simulink model "test2"  (R2015a)
settings: Solver=ode45  StartTime=0.0  StopTime=100000  RelTol=1e-3
InitFcn:
  | %% DSPBuilder Start
  | alt_dspbuilder_update_model(bdroot)
  | %% DSPBuilder End
libraries: allblocks_alteradspbuilder2 x988
(part 1 of 12)
settings Model: Creator=ASUS  LastModifiedBy=ASUS

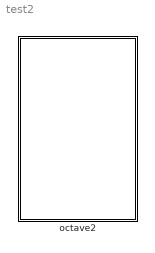
== system test2 ==
  octave2 : Subsystem

== system test2/octave2 ==
  AltBus : allblocks_alteradspbuilder2/AltBus  BusType=Unsigned Integer  bwl=128  bwr=0  saturate=off  floatingPointInput=on  floatingPointOutput=on  logOutputs=off  logFile=C:\Users\ASUS\Desktop\sift_fpga_final\Octave_2\tb_test2\test2_octave2_AltBus.fixedpointlog
  AltBus1 : allblocks_alteradspbuilder2/AltBus  BusType=Unsigned Fractional  bwl=8  bwr=16  saturate=off  floatingPointInput=on  floatingPointOutput=on  logOutputs=off  logFile=C:\Users\ASUS\Desktop\sift_fpga_final\Octave_2\tb_test2\test2_octave2_AltBus1.fixedpointlog
  AltBus2 : allblocks_alteradspbuilder2/AltBus  BusType=Unsigned Integer  bwl=10  bwr=16  saturate=off  floatingPointInput=on  floatingPointOutput=on  logOutputs=off  logFile=C:\Users\ASUS\Desktop\sift_fpga_final\Octave_2\tb_test2\test2_octave2_AltBus2.fixedpointlog
  AltBus3 : allblocks_alteradspbuilder2/AltBus  BusType=Unsigned Integer  bwl=8  bwr=0  saturate=off  floatingPointInput=on  floatingPointOutput=on  logOutputs=off  logFile=C:\Users\ASUS\Desktop\sift_fpga_final\Octave_2\tb_test2\test2_octave2_AltBus3.fixedpointlog
  Bus_Concatenation : Subsystem
  From Workspace : FromWorkspace  VariableName=pixel_in  SampleTime=0
  From Workspace1 : FromWorkspace  VariableName=valid_in  SampleTime=0
  From Workspace2 : FromWorkspace  VariableName=sof_in  SampleTime=0
  From Workspace3 : FromWorkspace  VariableName=eof_in  SampleTime=0
  GradOrien : Subsystem
  Line_buff_11x11 : Subsystem
  descriptor : Subsystem
  hist_bin : Subsystem
  scale_space : Subsystem
  sink_validIn : allblocks_alteradspbuilder2/Input  iofile=C:\Users\ASUS\Desktop\sift_fpga_final\Octave_2\tb_test2\test2_octave2_sink%5FvalidIn.salt  BusType=Single Bit  bwl=8  bwr=0  SpecifyClock=off  PORTTYPE=Input  externalType=Inferred  allowFloatingPointOverride=on  logOutputs=off
  sink_validIn1 : allblocks_alteradspbuilder2/Input  iofile=C:\Users\ASUS\Desktop\sift_fpga_final\Octave_2\tb_test2\test2_octave2_sink%5FvalidIn1.salt  BusType=Single Bit  bwl=8  bwr=0  SpecifyClock=off  PORTTYPE=Input  externalType=Inferred  allowFloatingPointOverride=on  logOutputs=off
  sink_validIn2 : allblocks_alteradspbuilder2/Input  iofile=C:\Users\ASUS\Desktop\sift_fpga_final\Octave_2\tb_test2\test2_octave2_sink%5FvalidIn2.salt  BusType=Single Bit  bwl=8  bwr=0  SpecifyClock=off  PORTTYPE=Input  externalType=Inferred  allowFloatingPointOverride=on  logOutputs=off
  sink_validIn3 : allblocks_alteradspbuilder2/Input  iofile=C:\Users\ASUS\Desktop\sift_fpga_final\Octave_2\tb_test2\test2_octave2_sink%5FvalidIn3.salt  BusType=Unsigned Integer  bwl=8  bwr=0  SpecifyClock=off  PORTTYPE=Input  externalType=Inferred  allowFloatingPointOverride=on  logOutputs=off
  wires:
  GradOrien/1(m_xy) -> AltBus2/1
  hist_bin/6(hist_bin6_out) -> Bus_Concatenation/6(bin6_in)
  hist_bin/8(hist_bin8_out) -> Bus_Concatenation/8(bin8_in)
  [valid_in] -> scale_space/2(valid_in)
  scale_space/1(scale2) -> AltBus1/1
  [valid_in] -> GradOrien/2(clken)
  [pixel_in] -> scale_space/1(data_in)
  [valid_in] -> hist_bin/3(clken)
  GradOrien/2(orien) -> AltBus3/1
  hist_bin/7(hist_bin7_out) -> Bus_Concatenation/7(bin_in)
  Line_buff_11x11/9(Out1010) -> descriptor/9(data_in1010)
  Line_buff_11x11/1(Out00) -> descriptor/1(data_in00)
  Line_buff_11x11/6(Out510) -> descriptor/6(data_in510)
  Line_buff_11x11/3(Out010) -> descriptor/3(data_in010)
  Line_buff_11x11/7(Out100) -> descriptor/7(data_in100)
  hist_bin/5(hist_bin5_out) -> Bus_Concatenation/5(bin5_in)
  hist_bin/3(hist_bin3_out) -> Bus_Concatenation/3(biin3_in)
  hist_bin/2(hist_bin2_out) -> Bus_Concatenation/2(bin2_in)
  Line_buff_11x11/2(Out05) -> descriptor/2(data_in05)
  hist_bin/1(hist_bin1_out) -> Bus_Concatenation/1(bin1_in)
  [valid_in] -> Line_buff_11x11/2(clken)
  hist_bin/4(hist_bin4_out) -> Bus_Concatenation/4(bin4_in)
  Line_buff_11x11/4(Out50) -> descriptor/4(data_in50)
  Line_buff_11x11/5(Out55) -> descriptor/5(data_in55)
  Bus_Concatenation/1(hist_bin) -> AltBus/1
  Line_buff_11x11/8(Out105) -> descriptor/8(data_in105)
  From Workspace2/1 -> sink_validIn1/1
  From Workspace/1 -> sink_validIn3/1
  From Workspace3/1 -> sink_validIn/1
  From Workspace1/1 -> sink_validIn2/1
  sink_validIn/1 -> [eof_in]
  sink_validIn1/1 -> [sof_in]
  sink_validIn2/1 -> [valid_in]
  sink_validIn3/1 -> [pixel_in]
  AltBus/1 -> Line_buff_11x11/1(dataIn)
  AltBus1/1 -> GradOrien/1(data_in)
  AltBus2/1 -> hist_bin/1(m_xy_In)
  AltBus3/1 -> hist_bin/2(orien_In)

== system test2/octave2/Bus_Concatenation ==
  bin1_in : Inport
  bin2_in : Inport  Port=2
  biin3_in : Inport  Port=3
  bin4_in : Inport  Port=4
  bin5_in : Inport  Port=5
  bin6_in : Inport  Port=6
  bin_in : Inport  Port=7
  bin8_in : Inport  Port=8
  Bus Concatenation{,1..3} (4 alike) : allblocks_alteradspbuilder2/Bus Concatenation  isSigned=off  awidth=16  bwidth=16  pipeline_display=0
  Bus Concatenation7 : allblocks_alteradspbuilder2/Bus Concatenation  isSigned=off  awidth=32  bwidth=32  pipeline_display=0
  Bus Concatenation8 : allblocks_alteradspbuilder2/Bus Concatenation  isSigned=off  awidth=32  bwidth=32  pipeline_display=0
  Bus Concatenation9 : allblocks_alteradspbuilder2/Bus Concatenation  isSigned=off  awidth=64  bwidth=64  pipeline_display=0
  To Workspace : ToWorkspace  VariableName=bin1  SaveFormat=Timeseries  SampleTime=-1
  hist_bin : Outport
  wires:
  bin1_in/1 -> [bin1]
  bin2_in/1 -> [bin2]
  biin3_in/1 -> [bin3]
  bin4_in/1 -> [bin4]
  bin5_in/1 -> [bin5]
  bin6_in/1 -> [bin6]
  bin_in/1 -> [bin7]
  bin8_in/1 -> [bin8]
  Bus Concatenation/1 -> Bus Concatenation8/2
  [bin6] -> Bus Concatenation1/2
  Bus Concatenation1/1 -> Bus Concatenation8/1
  [bin8] -> Bus Concatenation/2
  [bin5] -> Bus Concatenation1/1
  [bin7] -> Bus Concatenation/1
  Bus Concatenation9/1 -> To Workspace/1, hist_bin/1
  [bin4] -> Bus Concatenation2/2
  [bin3] -> Bus Concatenation2/1
  [bin2] -> Bus Concatenation3/2
  [bin1] -> Bus Concatenation3/1
  Bus Concatenation3/1 -> Bus Concatenation7/1
  Bus Concatenation2/1 -> Bus Concatenation7/2
  Bus Concatenation7/1 -> Bus Concatenation9/1
  Bus Concatenation8/1 -> Bus Concatenation9/2

== system test2/octave2/GradOrien ==
  data_in : Inport
  clken : Inport  Port=2
  lineBuff_3x3 : Subsystem
  sub_GradOrian : Subsystem
  m_xy : Outport
  orien : Outport  Port=2
  wires:
  sub_GradOrian/1(orien) -> orien/1
  clken/1 -> sub_GradOrian/5(clken), lineBuff_3x3/2(clken)
  data_in/1 -> lineBuff_3x3/1(dataIn)
  sub_GradOrian/2(m_xy) -> m_xy/1
  lineBuff_3x3/1(Out01) -> sub_GradOrian/1(L_y_add_1)
  lineBuff_3x3/4(Out21) -> sub_GradOrian/4(L_y_sub_1)
  lineBuff_3x3/3(Out12) -> sub_GradOrian/3(L_x_sub_1)
  lineBuff_3x3/2(Out10) -> sub_GradOrian/2(L_x_add_1)

== system test2/octave2/Line_buff_11x11 ==
  dataIn : Inport
  clken : Inport  Port=2
  Memory Delay1 : allblocks_alteradspbuilder2/Memory Delay  BusType=Unsigned Integer  bwl=128  bwr=0  pipeline=1  pipeline_display=1  ram_type=AUTO  use_ena=on  use_sclr=off  allowFloatingPointOverride=on  logOutputs=off  logFile=C:\Users\ASUS\Desktop\sift_fpga_final\Octave_2\tb_test2\test2_octave2_Line%5Fbuff%5F11x11_Memory+Delay1.fixedpointlog
  Memory Delay11 : allblocks_alteradspbuilder2/Memory Delay  BusType=Unsigned Integer  bwl=128  bwr=0  pipeline=630  pipeline_display=630  ram_type=AUTO  use_ena=on  use_sclr=off  allowFloatingPointOverride=on  logOutputs=off  logFile=C:\Users\ASUS\Desktop\sift_fpga_final\Octave_2\tb_test2\test2_octave2_Line%5Fbuff%5F11x11_Memory+Delay11.fixedpointlog
  Memory Delay12 : allblocks_alteradspbuilder2/Memory Delay  BusType=Unsigned Integer  bwl=128  bwr=0  pipeline=5  pipeline_display=5  ram_type=AUTO  use_ena=on  use_sclr=off  allowFloatingPointOverride=on  logOutputs=off  logFile=C:\Users\ASUS\Desktop\sift_fpga_final\Octave_2\tb_test2\test2_octave2_Line%5Fbuff%5F11x11_Memory+Delay12.fixedpointlog
  Memory Delay13 : allblocks_alteradspbuilder2/Memory Delay  BusType=Unsigned Integer  bwl=128  bwr=0  pipeline=5  pipeline_display=5  ram_type=AUTO  use_ena=on  use_sclr=off  allowFloatingPointOverride=on  logOutputs=off  logFile=C:\Users\ASUS\Desktop\sift_fpga_final\Octave_2\tb_test2\test2_octave2_Line%5Fbuff%5F11x11_Memory+Delay13.fixedpointlog
  Memory Delay15 : allblocks_alteradspbuilder2/Memory Delay  BusType=Unsigned Integer  bwl=128  bwr=0  pipeline=630  pipeline_display=630  ram_type=AUTO  use_ena=on  use_sclr=off  allowFloatingPointOverride=on  logOutputs=off  logFile=C:\Users\ASUS\Desktop\sift_fpga_final\Octave_2\tb_test2\test2_octave2_Line%5Fbuff%5F11x11_Memory+Delay15.fixedpointlog
  Memory Delay16 : allblocks_alteradspbuilder2/Memory Delay  BusType=Unsigned Integer  bwl=128  bwr=0  pipeline=5  pipeline_display=5  ram_type=AUTO  use_ena=on  use_sclr=off  allowFloatingPointOverride=on  logOutputs=off  logFile=C:\Users\ASUS\Desktop\sift_fpga_final\Octave_2\tb_test2\test2_octave2_Line%5Fbuff%5F11x11_Memory+Delay16.fixedpointlog
  Memory Delay17 : allblocks_alteradspbuilder2/Memory Delay  BusType=Unsigned Integer  bwl=128  bwr=0  pipeline=5  pipeline_display=5  ram_type=AUTO  use_ena=on  use_sclr=off  allowFloatingPointOverride=on  logOutputs=off  logFile=C:\Users\ASUS\Desktop\sift_fpga_final\Octave_2\tb_test2\test2_octave2_Line%5Fbuff%5F11x11_Memory+Delay17.fixedpointlog
  Memory Delay18 : allblocks_alteradspbuilder2/Memory Delay  BusType=Unsigned Integer  bwl=128  bwr=0  pipeline=640*4  pipeline_display=2560  ram_type=AUTO  use_ena=on  use_sclr=off  allowFloatingPointOverride=on  logOutputs=off  logFile=C:\Users\ASUS\Desktop\sift_fpga_final\Octave_2\tb_test2\test2_octave2_Line%5Fbuff%5F11x11_Memory+Delay18.fixedpointlog
  Memory Delay5 : allblocks_alteradspbuilder2/Memory Delay  BusType=Unsigned Integer  bwl=128  bwr=0  pipeline=5  pipeline_display=5  ram_type=AUTO  use_ena=on  use_sclr=off  allowFloatingPointOverride=on  logOutputs=off  logFile=C:\Users\ASUS\Desktop\sift_fpga_final\Octave_2\tb_test2\test2_octave2_Line%5Fbuff%5F11x11_Memory+Delay5.fixedpointlog
  Memory Delay6 : allblocks_alteradspbuilder2/Memory Delay  BusType=Unsigned Integer  bwl=128  bwr=0  pipeline=5  pipeline_display=5  ram_type=AUTO  use_ena=on  use_sclr=off  allowFloatingPointOverride=on  logOutputs=off  logFile=C:\Users\ASUS\Desktop\sift_fpga_final\Octave_2\tb_test2\test2_octave2_Line%5Fbuff%5F11x11_Memory+Delay6.fixedpointlog
  Memory Delay7 : allblocks_alteradspbuilder2/Memory Delay  BusType=Unsigned Integer  bwl=128  bwr=0  pipeline=640*4  pipeline_display=2560  ram_type=AUTO  use_ena=on  use_sclr=off  allowFloatingPointOverride=on  logOutputs=off  logFile=C:\Users\ASUS\Desktop\sift_fpga_final\Octave_2\tb_test2\test2_octave2_Line%5Fbuff%5F11x11_Memory+Delay7.fixedpointlog
  Out00 : Outport
  Out05 : Outport  Port=2
  Out010 : Outport  Port=3
  Out50 : Outport  Port=4
  Out55 : Outport  Port=5
  Out510 : Outport  Port=6
  Out100 : Outport  Port=7
  Out105 : Outport  Port=8
  Out1010 : Outport  Port=9
  wires:
  [clken] -> Memory Delay11/2
  [clken] -> Memory Delay17/2
  [clken] -> Memory Delay6/2
  Memory Delay6/1 -> [data_010], Memory Delay7/1
  [clken] -> Memory Delay18/2
  Memory Delay18/1 -> Memory Delay15/1
  Memory Delay13/1 -> Memory Delay18/1, [data_510]
  [clken] -> Memory Delay15/2
  [clken] -> Memory Delay16/2
  Memory Delay17/1 -> [data_1010]
  Memory Delay16/1 -> Memory Delay17/1, [data_105]
  Memory Delay15/1 -> Memory Delay16/1, [data_100]
  [clken] -> Memory Delay7/2
  [clken] -> Memory Delay12/2
  Memory Delay11/1 -> Memory Delay12/1, [data_50]
  Memory Delay12/1 -> Memory Delay13/1, [data_55]
  Memory Delay7/1 -> Memory Delay11/1
  [clken] -> Memory Delay13/2
  [data_55] -> Out55/1
  [data_010] -> Out010/1
  [data_05] -> Out05/1
  clken/1 -> [clken]
  [data_00] -> Out00/1
  [data_50] -> Out50/1
  [data_100] -> Out100/1
  [data_510] -> Out510/1
  [data_1010] -> Out1010/1
  dataIn/1 -> [data_in]
  [data_105] -> Out105/1
  [clken] -> Memory Delay5/2
  Memory Delay1/1 -> Memory Delay5/1, [data_00]
  [clken] -> Memory Delay1/2
  [data_in] -> Memory Delay1/1
  Memory Delay5/1 -> Memory Delay6/1, [data_05]

== system test2/octave2/descriptor ==
  data_in00 : Inport
  data_in05 : Inport  Port=2
  data_in010 : Inport  Port=3
  data_in50 : Inport  Port=4
  data_in55 : Inport  Port=5
  data_in510 : Inport  Port=6
  data_in100 : Inport  Port=7
  data_in105 : Inport  Port=8
  data_in1010 : Inport  Port=9
  AltBus : allblocks_alteradspbuilder2/AltBus  BusType=Unsigned Integer  bwl=128*9  bwr=0  saturate=off  floatingPointInput=on  floatingPointOutput=on  logOutputs=off  logFile=C:\Users\ASUS\Desktop\sift_fpga_final\Octave_2\tb_test2\test2_octave2_descriptor_AltBus.fixedpointlog
  BusSplitter : Subsystem
  Multiplexer3 : allblocks_alteradspbuilder2/Multiplexer  numInputs=8  pipeline=0  oneHot=off  pipeline_display=0  use_ena=off  use_aclr=off  allowFloatingPointOverride=on  logOutputs=off  logFile=C:\Users\ASUS\Desktop\sift_fpga_final\Octave_2\tb_test2\test2_octave2_descriptor_Multiplexer3.fixedpointlog
  To Workspace1 : ToWorkspace  VariableName=descriptor  SaveFormat=Timeseries  SampleTime=-1
  To Workspace4 : ToWorkspace  VariableName=bin55  SaveFormat=Timeseries  SampleTime=-1
  To Workspace5 : ToWorkspace  VariableName=binmax  SaveFormat=Timeseries  SampleTime=-1
  descriptor : Subsystem
  findMax : Subsystem
  wires:
  [hist_105] -> descriptor/8(data_in8)
  [hist_100] -> descriptor/7(data_in7)
  [hist_510] -> descriptor/6(data_in6)
  [hist_55] -> descriptor/5(data_in5)
  [hist_1010] -> descriptor/9(data_in9)
  descriptor/1(descriptor1) -> Multiplexer3/2
  [hist_05] -> descriptor/2(data_in2)
  [hist_010] -> descriptor/3(data_in3)
  [hist_50] -> descriptor/4(data_in4)
  descriptor/5(descriptor5) -> Multiplexer3/6
  descriptor/4(descriptor4) -> Multiplexer3/5
  [hist_00] -> descriptor/1(data_in1)
  descriptor/7(descriptor7) -> Multiplexer3/8
  descriptor/8(descriptor8) -> Multiplexer3/9
  descriptor/2(descriptor2) -> Multiplexer3/3
  descriptor/3(descriptor3) -> Multiplexer3/4
  descriptor/6(descriptor6) -> Multiplexer3/7
  BusSplitter/3(bin3) -> findMax/3(bin3)
  data_in00/1 -> [hist_00]
  data_in50/1 -> [hist_50]
  BusSplitter/1(bin1) -> findMax/1(bin1)
  data_in100/1 -> [hist_100]
  data_in010/1 -> [hist_010]
  data_in105/1 -> [hist_105]
  [hist_55] -> To Workspace4/1, BusSplitter/1(data_in)
  data_in510/1 -> [hist_510]
  data_in1010/1 -> [hist_1010]
  BusSplitter/8(bin8) -> findMax/8(bin8)
  data_in55/1 -> [hist_55]
  BusSplitter/4(bin4) -> findMax/4(bin4)
  BusSplitter/2(bin2) -> findMax/2(bin2)
  data_in05/1 -> [hist_05]
  BusSplitter/5(bin5) -> findMax/5(bin5)
  BusSplitter/7(bin7) -> findMax/7(bin7)
  BusSplitter/6(bin6) -> findMax/6(bin6)
  AltBus/1 -> [descriptor]
  findMax/1(bin_max) -> To Workspace5/1, Multiplexer3/1
  Multiplexer3/1 -> To Workspace1/1, AltBus/1

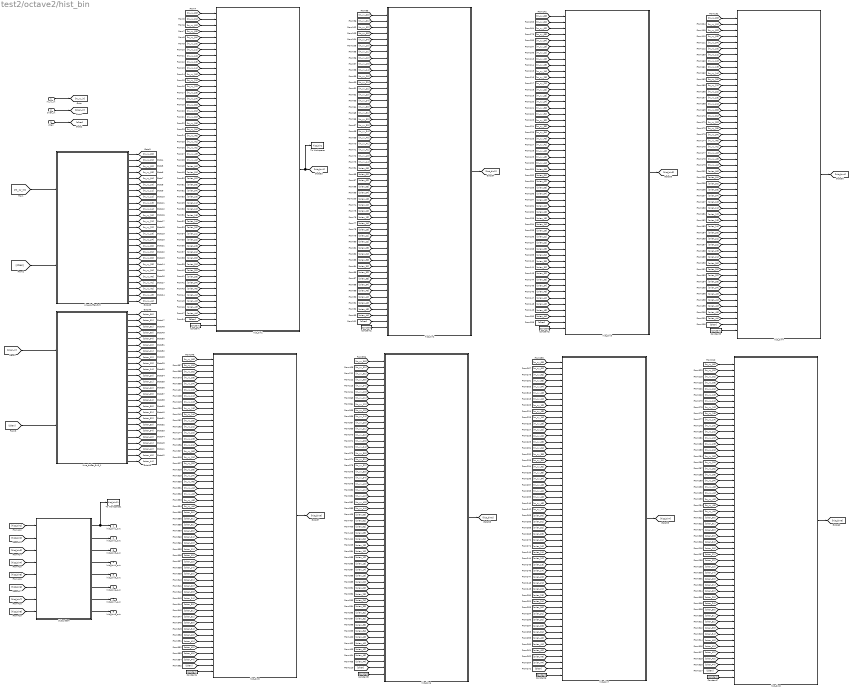
== system test2/octave2/hist_bin ==
  m_xy_In : Inport
  orien_In : Inport  Port=2
  clken : Inport  Port=3
  Constant : allblocks_alteradspbuilder2/Constant  mask_cst=1  BusType=Unsigned Integer  bwl=8  bwr=0  roundMode=Truncate  satMode=Wrap  SpecifyClock=off  allowFloatingPointOverride=on  logOutputs=off  logFile=C:\Users\ASUS\Desktop\sift_fpga_final\Octave_2\tb_test2\test2_octave2_hist%5Fbin_Constant.fixedpointlog
  Constant1 : allblocks_alteradspbuilder2/Constant  mask_cst=2  BusType=Unsigned Integer  bwl=8  bwr=0  roundMode=Truncate  satMode=Wrap  SpecifyClock=off  allowFloatingPointOverride=on  logOutputs=off  logFile=C:\Users\ASUS\Desktop\sift_fpga_final\Octave_2\tb_test2\test2_octave2_hist%5Fbin_Constant1.fixedpointlog
  Constant2 : allblocks_alteradspbuilder2/Constant  mask_cst=3  BusType=Unsigned Integer  bwl=8  bwr=0  roundMode=Truncate  satMode=Wrap  SpecifyClock=off  allowFloatingPointOverride=on  logOutputs=off  logFile=C:\Users\ASUS\Desktop\sift_fpga_final\Octave_2\tb_test2\test2_octave2_hist%5Fbin_Constant2.fixedpointlog
  Constant3 : allblocks_alteradspbuilder2/Constant  mask_cst=4  BusType=Unsigned Integer  bwl=8  bwr=0  roundMode=Truncate  satMode=Wrap  SpecifyClock=off  allowFloatingPointOverride=on  logOutputs=off  logFile=C:\Users\ASUS\Desktop\sift_fpga_final\Octave_2\tb_test2\test2_octave2_hist%5Fbin_Constant3.fixedpointlog
  Constant4 : allblocks_alteradspbuilder2/Constant  mask_cst=5  BusType=Unsigned Integer  bwl=8  bwr=0  roundMode=Truncate  satMode=Wrap  SpecifyClock=off  allowFloatingPointOverride=on  logOutputs=off  logFile=C:\Users\ASUS\Desktop\sift_fpga_final\Octave_2\tb_test2\test2_octave2_hist%5Fbin_Constant4.fixedpointlog
  Constant5 : allblocks_alteradspbuilder2/Constant  mask_cst=6  BusType=Unsigned Integer  bwl=8  bwr=0  roundMode=Truncate  satMode=Wrap  SpecifyClock=off  allowFloatingPointOverride=on  logOutputs=off  logFile=C:\Users\ASUS\Desktop\sift_fpga_final\Octave_2\tb_test2\test2_octave2_hist%5Fbin_Constant5.fixedpointlog
  Constant6 : allblocks_alteradspbuilder2/Constant  mask_cst=7  BusType=Unsigned Integer  bwl=8  bwr=0  roundMode=Truncate  satMode=Wrap  SpecifyClock=off  allowFloatingPointOverride=on  logOutputs=off  logFile=C:\Users\ASUS\Desktop\sift_fpga_final\Octave_2\tb_test2\test2_octave2_hist%5Fbin_Constant6.fixedpointlog
  Constant7 : allblocks_alteradspbuilder2/Constant  mask_cst=8  BusType=Unsigned Integer  bwl=8  bwr=0  roundMode=Truncate  satMode=Wrap  SpecifyClock=off  allowFloatingPointOverride=on  logOutputs=off  logFile=C:\Users\ASUS\Desktop\sift_fpga_final\Octave_2\tb_test2\test2_octave2_hist%5Fbin_Constant7.fixedpointlog
  Line_buffer_5x5 : Subsystem
  Line_buffer_5x5_1 : Subsystem
  Subsystem : Subsystem
  To Workspace : ToWorkspace  VariableName=hist_bin1  SaveFormat=Timeseries  SampleTime=-1
  To Workspace1 : ToWorkspace  VariableName=hist_bin11  SaveFormat=Timeseries  SampleTime=-1
  hist_bin1 : Subsystem
  hist_bin2 : Subsystem
  hist_bin3 : Subsystem
  hist_bin4 : Subsystem
  hist_bin5 : Subsystem
  hist_bin6 : Subsystem
  hist_bin7 : Subsystem
  hist_bin8 : Subsystem
  hist_bin1_out : Outport
  hist_bin2_out : Outport  Port=2
  hist_bin3_out : Outport  Port=3
  hist_bin4_out : Outport  Port=4
  hist_bin5_out : Outport  Port=5
  hist_bin6_out : Outport  Port=6
  hist_bin7_out : Outport  Port=7
  hist_bin8_out : Outport  Port=8
  wires:
  [hist_bin7] -> Subsystem/7(hist_in_bin7)
  [m_xy_in] -> Line_buffer_5x5/1(dataIn)
  [clken] -> Line_buffer_5x5/2(clken)
  [clken] -> Line_buffer_5x5_1/2(clken)
  [orien_in] -> Line_buffer_5x5_1/1(dataIn)
  clken/1 -> [clken]
  Line_buffer_5x5_1/21(Out40) -> [orien_40]
  Line_buffer_5x5_1/19(Out33) -> [orien_33]
  Line_buffer_5x5_1/8(Out12) -> [orien_12]
  Line_buffer_5x5_1/14(Out23) -> [orien_23]
  Line_buffer_5x5_1/18(Out32) -> [orien_32]
  Line_buffer_5x5_1/20(Out34) -> [orien_34]
  Line_buffer_5x5_1/2(Out01) -> [orien_01]
  Line_buffer_5x5_1/7(Out11) -> [orien_11]
  Line_buffer_5x5_1/11(Out20) -> [orien_20]
  Line_buffer_5x5_1/13(Out22) -> [orien_22]
  Line_buffer_5x5_1/17(Out31) -> [orien_31]
  Line_buffer_5x5_1/25(Out44) -> [orien_44]
  Line_buffer_5x5_1/3(Out02) -> [orien_02]
  Line_buffer_5x5_1/5(Out04) -> [orien_04]
  Line_buffer_5x5_1/23(Out42) -> [orien_42]
  Line_buffer_5x5_1/24(Out43) -> [orien_43]
  Line_buffer_5x5_1/6(Out10) -> [orien_10]
  Line_buffer_5x5_1/1(Out00) -> [orien_00]
  Line_buffer_5x5_1/22(Out41) -> [orien_41]
  Line_buffer_5x5_1/15(Out24) -> [orien_24]
  Line_buffer_5x5_1/4(Out03) -> [orien_03]
  Line_buffer_5x5_1/9(Out13) -> [orien_13]
  Line_buffer_5x5_1/10(Out14) -> [orien_14]
  Line_buffer_5x5_1/12(Out21) -> [orien_21]
  Line_buffer_5x5_1/16(Out30) -> [orien_30]
  Line_buffer_5x5/24(Out43) -> [m_xy_43]
  Line_buffer_5x5/21(Out40) -> [m_xy_40]
  Line_buffer_5x5/23(Out42) -> [m_xy_42]
  Line_buffer_5x5/22(Out41) -> [m_xy_41]
  Line_buffer_5x5/25(Out44) -> [m_xy_44]
  Line_buffer_5x5/12(Out21) -> [m_xy_21]
  Line_buffer_5x5/15(Out24) -> [m_xy_24]
  Line_buffer_5x5/19(Out33) -> [m_xy_33]
  Line_buffer_5x5/18(Out32) -> [m_xy_32]
  Line_buffer_5x5/13(Out22) -> [m_xy_22]
  Line_buffer_5x5/11(Out20) -> [m_xy_20]
  Line_buffer_5x5/16(Out30) -> [m_xy_30]
  Line_buffer_5x5/14(Out23) -> [m_xy_23]
  Line_buffer_5x5/17(Out31) -> [m_xy_31]
  Line_buffer_5x5/20(Out34) -> [m_xy_34]
  [hist_bin1] -> Subsystem/1(hist_in_bin1)
  Line_buffer_5x5/1(Out00) -> [m_xy_00]
  [m_xy_04] -> hist_bin1/5(Mxy_In04)
  Line_buffer_5x5/2(Out01) -> [m_xy_01]
  hist_bin1/1(bin_out) -> To Workspace/1, [hist_bin1]
  [m_xy_10] -> hist_bin1/6(Mxy_In10)
  Line_buffer_5x5/9(Out13) -> [m_xy_13]
  [m_xy_13] -> hist_bin1/9(Mxy_In13)
  Line_buffer_5x5/10(Out14) -> [m_xy_14]
  Line_buffer_5x5/6(Out10) -> [m_xy_10]
  Line_buffer_5x5/7(Out11) -> [m_xy_11]
  [m_xy_11] -> hist_bin1/7(Mxy_In11)
  [m_xy_12] -> hist_bin1/8(Mxy_In12)
  Line_buffer_5x5/8(Out12) -> [m_xy_12]
  [m_xy_14] -> hist_bin1/10(Mxy_In14)
  [m_xy_22] -> hist_bin1/13(Mxy_In22)
  [m_xy_40] -> hist_bin1/21(Mxy_In40)
  [m_xy_43] -> hist_bin1/24(Mxy_In43)
  [m_xy_42] -> hist_bin1/23(Mxy_In42)
  [m_xy_44] -> hist_bin1/25(Mxy_In44)
  [m_xy_24] -> hist_bin1/15(Mxy_In24)
  [m_xy_21] -> hist_bin1/12(Mxy_In21)
  [m_xy_20] -> hist_bin1/11(Mxy_In20)
  [m_xy_23] -> hist_bin1/14(Mxy_In23)
  [m_xy_41] -> hist_bin1/22(Mxy_In41)
  [m_xy_01] -> hist_bin1/2(Mxy_In01)
  Line_buffer_5x5/4(Out03) -> [m_xy_03]
  Line_buffer_5x5/5(Out04) -> [m_xy_04]
  Line_buffer_5x5/3(Out02) -> [m_xy_02]
  [m_xy_31] -> hist_bin1/17(Mxy_In31)
  [m_xy_30] -> hist_bin1/16(Mxy_In30)
  [m_xy_34] -> hist_bin1/20(Mxy_In34)
  [m_xy_33] -> hist_bin1/19(Mxy_In33)
  [m_xy_32] -> hist_bin1/18(Mxy_In32)
  [m_xy_03] -> hist_bin1/4(Mxy_In03)
  [m_xy_02] -> hist_bin1/3(Mxy_In02)
  [hist_bin3] -> Subsystem/3(hist_in_bin3)
  [hist_bin4] -> Subsystem/4(hist_in_bin4)
  [orien_10] -> hist_bin1/31(Orien_In10)
  [orien_42] -> hist_bin1/48(Orien_In42)
  [orien_01] -> hist_bin1/27(Orien_In01)
  [orien_20] -> hist_bin1/36(Orien_In20)
  [orien_31] -> hist_bin1/42(Orien_In31)
  [orien_33] -> hist_bin1/44(Orien_In33)
  [orien_21] -> hist_bin1/37(Orien_In21)
  [orien_24] -> hist_bin1/40(Orien_In24)
  [orien_03] -> hist_bin1/29(Orien_In03)
  [orien_30] -> hist_bin1/41(Orien_In30)
  [orien_12] -> hist_bin1/33(Orien_In12)
  [orien_23] -> hist_bin1/39(Orien_In23)
  [orien_32] -> hist_bin1/43(Orien_In32)
  [orien_41] -> hist_bin1/47(Orien_In41)
  [orien_43] -> hist_bin1/49(Orien_In43)
  [orien_02] -> hist_bin1/28(Orien_In02)
  [orien_00] -> hist_bin1/26(Orien_In00)
  [orien_11] -> hist_bin1/32(Orien_In11)
  [orien_34] -> hist_bin1/45(Orien_In34)
  [orien_22] -> hist_bin1/38(Orien_In22)
  [orien_04] -> hist_bin1/30(Orien_In04)
  [orien_14] -> hist_bin1/35(Orien_In14)
  [orien_44] -> hist_bin1/50(Orien_In44)
  [orien_13] -> hist_bin1/34(Orien_In13)
  [orien_40] -> hist_bin1/46(Orien_In40)
  [clken] -> hist_bin1/51(clken)
  Constant/1 -> hist_bin1/52(bin_in)
  [m_xy_02] -> hist_bin2/3(Mxy_In02)
  [m_xy_04] -> hist_bin2/5(Mxy_In04)
  [m_xy_10] -> hist_bin2/6(Mxy_In10)
  [m_xy_23] -> hist_bin2/14(Mxy_In23)
  [m_xy_31] -> hist_bin2/17(Mxy_In31)
  [m_xy_30] -> hist_bin2/16(Mxy_In30)
  [m_xy_12] -> hist_bin2/8(Mxy_In12)
  [m_xy_32] -> hist_bin2/18(Mxy_In32)
  [m_xy_13] -> hist_bin2/9(Mxy_In13)
  [m_xy_33] -> hist_bin2/19(Mxy_In33)
  [m_xy_41] -> hist_bin2/22(Mxy_In41)
  [m_xy_01] -> hist_bin2/2(Mxy_In01)
  [m_xy_14] -> hist_bin2/10(Mxy_In14)
  [m_xy_40] -> hist_bin2/21(Mxy_In40)
  [m_xy_43] -> hist_bin2/24(Mxy_In43)
  [m_xy_20] -> hist_bin2/11(Mxy_In20)
  [m_xy_22] -> hist_bin2/13(Mxy_In22)
  [m_xy_24] -> hist_bin2/15(Mxy_In24)
  [m_xy_34] -> hist_bin2/20(Mxy_In34)
  [m_xy_03] -> hist_bin2/4(Mxy_In03)
  [m_xy_00] -> hist_bin2/1(Mxy_In00)
  [m_xy_11] -> hist_bin2/7(Mxy_In11)
  [m_xy_21] -> hist_bin2/12(Mxy_In21)
  [orien_31] -> hist_bin2/42(Orien_In31)
  [orien_34] -> hist_bin2/45(Orien_In34)
  [m_xy_42] -> hist_bin2/23(Mxy_In42)
  [orien_01] -> hist_bin2/27(Orien_In01)
  [orien_00] -> hist_bin2/26(Orien_In00)
  [orien_04] -> hist_bin2/30(Orien_In04)
  [orien_13] -> hist_bin2/34(Orien_In13)
  [orien_20] -> hist_bin2/36(Orien_In20)
  [orien_24] -> hist_bin2/40(Orien_In24)
  [orien_33] -> hist_bin2/44(Orien_In33)
  [orien_32] -> hist_bin2/43(Orien_In32)
  [orien_41] -> hist_bin2/47(Orien_In41)
  [orien_11] -> hist_bin2/32(Orien_In11)
  [orien_21] -> hist_bin2/37(Orien_In21)
  [orien_14] -> hist_bin2/35(Orien_In14)
  [orien_22] -> hist_bin2/38(Orien_In22)
  [orien_23] -> hist_bin2/39(Orien_In23)
  [orien_02] -> hist_bin2/28(Orien_In02)
  [orien_10] -> hist_bin2/31(Orien_In10)
  [orien_12] -> hist_bin2/33(Orien_In12)
  [orien_30] -> hist_bin2/41(Orien_In30)
  [m_xy_44] -> hist_bin2/25(Mxy_In44)
  [orien_03] -> hist_bin2/29(Orien_In03)
  [orien_40] -> hist_bin2/46(Orien_In40)
  [clken] -> hist_bin2/51(clken)
  hist_bin2/1(bin_out) -> [hist_bin2]
  [orien_42] -> hist_bin2/48(Orien_In42)
  [orien_44] -> hist_bin2/50(Orien_In44)
  [orien_43] -> hist_bin2/49(Orien_In43)
  Constant1/1 -> hist_bin2/52(bin_in)
  [m_xy_00] -> hist_bin1/1(Mxy_In00)
  Subsystem/4(bin4_out) -> hist_bin4_out/1
  Subsystem/3(bin3_out) -> hist_bin3_out/1
  [hist_bin8] -> Subsystem/8(hist_in_bin8)
  [hist_bin6] -> Subsystem/6(hist_in_bin6)
  [hist_bin5] -> Subsystem/5(hist_in_bin5)
  Subsystem/2(bin2_out) -> hist_bin2_out/1
  orien_In/1 -> [orien_in]
  m_xy_In/1 -> [m_xy_in]
  Subsystem/5(bin5_out) -> hist_bin5_out/1
  Subsystem/6(bin6_out) -> hist_bin6_out/1
  Subsystem/7(bin7_out) -> hist_bin7_out/1
  Subsystem/8(bin8_out) -> hist_bin8_out/1
  [hist_bin2] -> Subsystem/2(hist_in_bin2)
  [m_xy_04] -> hist_bin3/5(Mxy_In04)
  hist_bin3/1(bin_out) -> [hist_bin3]
  [m_xy_10] -> hist_bin3/6(Mxy_In10)
  [m_xy_13] -> hist_bin3/9(Mxy_In13)
  [m_xy_11] -> hist_bin3/7(Mxy_In11)
  [m_xy_12] -> hist_bin3/8(Mxy_In12)
  [m_xy_14] -> hist_bin3/10(Mxy_In14)
  [m_xy_22] -> hist_bin3/13(Mxy_In22)
  [m_xy_40] -> hist_bin3/21(Mxy_In40)
  [m_xy_43] -> hist_bin3/24(Mxy_In43)
  [m_xy_42] -> hist_bin3/23(Mxy_In42)
  [m_xy_44] -> hist_bin3/25(Mxy_In44)
  [m_xy_24] -> hist_bin3/15(Mxy_In24)
  [m_xy_21] -> hist_bin3/12(Mxy_In21)
  [m_xy_20] -> hist_bin3/11(Mxy_In20)
  [m_xy_23] -> hist_bin3/14(Mxy_In23)
  [m_xy_41] -> hist_bin3/22(Mxy_In41)
  [m_xy_01] -> hist_bin3/2(Mxy_In01)
  [m_xy_31] -> hist_bin3/17(Mxy_In31)
  [m_xy_30] -> hist_bin3/16(Mxy_In30)
  [m_xy_34] -> hist_bin3/20(Mxy_In34)
  [m_xy_33] -> hist_bin3/19(Mxy_In33)
  [m_xy_32] -> hist_bin3/18(Mxy_In32)
  [m_xy_03] -> hist_bin3/4(Mxy_In03)
  [m_xy_02] -> hist_bin3/3(Mxy_In02)
  [orien_10] -> hist_bin3/31(Orien_In10)
  [orien_42] -> hist_bin3/48(Orien_In42)
  [orien_01] -> hist_bin3/27(Orien_In01)
  [orien_20] -> hist_bin3/36(Orien_In20)
  [orien_31] -> hist_bin3/42(Orien_In31)
  [orien_33] -> hist_bin3/44(Orien_In33)
  [orien_21] -> hist_bin3/37(Orien_In21)
  [orien_24] -> hist_bin3/40(Orien_In24)
  [orien_03] -> hist_bin3/29(Orien_In03)
  [orien_30] -> hist_bin3/41(Orien_In30)
  [orien_12] -> hist_bin3/33(Orien_In12)
  [orien_23] -> hist_bin3/39(Orien_In23)
  [orien_32] -> hist_bin3/43(Orien_In32)
  [orien_41] -> hist_bin3/47(Orien_In41)
  [orien_43] -> hist_bin3/49(Orien_In43)
  [orien_02] -> hist_bin3/28(Orien_In02)
  [orien_00] -> hist_bin3/26(Orien_In00)
  [orien_11] -> hist_bin3/32(Orien_In11)
  [orien_34] -> hist_bin3/45(Orien_In34)
  [orien_22] -> hist_bin3/38(Orien_In22)
  [orien_04] -> hist_bin3/30(Orien_In04)
  [orien_14] -> hist_bin3/35(Orien_In14)
  [orien_44] -> hist_bin3/50(Orien_In44)
  [orien_13] -> hist_bin3/34(Orien_In13)
  [orien_40] -> hist_bin3/46(Orien_In40)
  [clken] -> hist_bin3/51(clken)
  Constant2/1 -> hist_bin3/52(bin_in)
  [m_xy_02] -> hist_bin4/3(Mxy_In02)
  [m_xy_04] -> hist_bin4/5(Mxy_In04)
  [m_xy_10] -> hist_bin4/6(Mxy_In10)
  [m_xy_23] -> hist_bin4/14(Mxy_In23)
  [m_xy_31] -> hist_bin4/17(Mxy_In31)
  [m_xy_30] -> hist_bin4/16(Mxy_In30)
  [m_xy_12] -> hist_bin4/8(Mxy_In12)
  [m_xy_32] -> hist_bin4/18(Mxy_In32)
  [m_xy_13] -> hist_bin4/9(Mxy_In13)
  [m_xy_33] -> hist_bin4/19(Mxy_In33)
  [m_xy_41] -> hist_bin4/22(Mxy_In41)
  [m_xy_01] -> hist_bin4/2(Mxy_In01)
  [m_xy_14] -> hist_bin4/10(Mxy_In14)
  [m_xy_40] -> hist_bin4/21(Mxy_In40)
  [m_xy_43] -> hist_bin4/24(Mxy_In43)
  [m_xy_20] -> hist_bin4/11(Mxy_In20)
  [m_xy_22] -> hist_bin4/13(Mxy_In22)
  [m_xy_24] -> hist_bin4/15(Mxy_In24)
  [m_xy_34] -> hist_bin4/20(Mxy_In34)
  [m_xy_03] -> hist_bin4/4(Mxy_In03)
  [m_xy_00] -> hist_bin4/1(Mxy_In00)
  [m_xy_11] -> hist_bin4/7(Mxy_In11)
  [m_xy_21] -> hist_bin4/12(Mxy_In21)
  [orien_31] -> hist_bin4/42(Orien_In31)
  [orien_34] -> hist_bin4/45(Orien_In34)
  [m_xy_42] -> hist_bin4/23(Mxy_In42)
  [orien_01] -> hist_bin4/27(Orien_In01)
  [orien_00] -> hist_bin4/26(Orien_In00)
  [orien_04] -> hist_bin4/30(Orien_In04)
  [orien_13] -> hist_bin4/34(Orien_In13)
  [orien_20] -> hist_bin4/36(Orien_In20)
  [orien_24] -> hist_bin4/40(Orien_In24)
  [orien_33] -> hist_bin4/44(Orien_In33)
  [orien_32] -> hist_bin4/43(Orien_In32)
  [orien_41] -> hist_bin4/47(Orien_In41)
  [orien_11] -> hist_bin4/32(Orien_In11)
  [orien_21] -> hist_bin4/37(Orien_In21)
  [orien_14] -> hist_bin4/35(Orien_In14)
  [orien_22] -> hist_bin4/38(Orien_In22)
  [orien_23] -> hist_bin4/39(Orien_In23)
  [orien_02] -> hist_bin4/28(Orien_In02)
  [orien_10] -> hist_bin4/31(Orien_In10)
  [orien_12] -> hist_bin4/33(Orien_In12)
  [orien_30] -> hist_bin4/41(Orien_In30)
  [m_xy_44] -> hist_bin4/25(Mxy_In44)
  [orien_03] -> hist_bin4/29(Orien_In03)
  [orien_40] -> hist_bin4/46(Orien_In40)
  [clken] -> hist_bin4/51(clken)
  hist_bin4/1(bin_out) -> [hist_bin4]
  [orien_42] -> hist_bin4/48(Orien_In42)
  [orien_44] -> hist_bin4/50(Orien_In44)
  [orien_43] -> hist_bin4/49(Orien_In43)
  Constant3/1 -> hist_bin4/52(bin_in)
  [m_xy_00] -> hist_bin3/1(Mxy_In00)
  [m_xy_04] -> hist_bin5/5(Mxy_In04)
  hist_bin5/1(bin_out) -> [hist_bin5]
  [m_xy_10] -> hist_bin5/6(Mxy_In10)
  [m_xy_13] -> hist_bin5/9(Mxy_In13)
  [m_xy_11] -> hist_bin5/7(Mxy_In11)
  [m_xy_12] -> hist_bin5/8(Mxy_In12)
  [m_xy_14] -> hist_bin5/10(Mxy_In14)
  [m_xy_22] -> hist_bin5/13(Mxy_In22)
  [m_xy_40] -> hist_bin5/21(Mxy_In40)
  [m_xy_43] -> hist_bin5/24(Mxy_In43)
  [m_xy_42] -> hist_bin5/23(Mxy_In42)
  [m_xy_44] -> hist_bin5/25(Mxy_In44)
  [m_xy_24] -> hist_bin5/15(Mxy_In24)
  [m_xy_21] -> hist_bin5/12(Mxy_In21)
  [m_xy_20] -> hist_bin5/11(Mxy_In20)
  [m_xy_23] -> hist_bin5/14(Mxy_In23)
  [m_xy_41] -> hist_bin5/22(Mxy_In41)
  [m_xy_01] -> hist_bin5/2(Mxy_In01)
  [m_xy_31] -> hist_bin5/17(Mxy_In31)
  [m_xy_30] -> hist_bin5/16(Mxy_In30)
  [m_xy_34] -> hist_bin5/20(Mxy_In34)
  [m_xy_33] -> hist_bin5/19(Mxy_In33)
  [m_xy_32] -> hist_bin5/18(Mxy_In32)
  [m_xy_03] -> hist_bin5/4(Mxy_In03)
  [m_xy_02] -> hist_bin5/3(Mxy_In02)
  [orien_10] -> hist_bin5/31(Orien_In10)
  [orien_42] -> hist_bin5/48(Orien_In42)
  [orien_01] -> hist_bin5/27(Orien_In01)
  [orien_20] -> hist_bin5/36(Orien_In20)
  [orien_31] -> hist_bin5/42(Orien_In31)
  [orien_33] -> hist_bin5/44(Orien_In33)
  [orien_21] -> hist_bin5/37(Orien_In21)
  [orien_24] -> hist_bin5/40(Orien_In24)
  [orien_03] -> hist_bin5/29(Orien_In03)
  [orien_30] -> hist_bin5/41(Orien_In30)
  [orien_12] -> hist_bin5/33(Orien_In12)
  [orien_23] -> hist_bin5/39(Orien_In23)
  [orien_32] -> hist_bin5/43(Orien_In32)
  [orien_41] -> hist_bin5/47(Orien_In41)
  [orien_43] -> hist_bin5/49(Orien_In43)
  [orien_02] -> hist_bin5/28(Orien_In02)
  [orien_00] -> hist_bin5/26(Orien_In00)
  [orien_11] -> hist_bin5/32(Orien_In11)
  [orien_34] -> hist_bin5/45(Orien_In34)
  [orien_22] -> hist_bin5/38(Orien_In22)
  [orien_04] -> hist_bin5/30(Orien_In04)
  [orien_14] -> hist_bin5/35(Orien_In14)
  [orien_44] -> hist_bin5/50(Orien_In44)
  [orien_13] -> hist_bin5/34(Orien_In13)
  [orien_40] -> hist_bin5/46(Orien_In40)
  [clken] -> hist_bin5/51(clken)
  Constant4/1 -> hist_bin5/52(bin_in)
  [m_xy_02] -> hist_bin6/3(Mxy_In02)
  [m_xy_04] -> hist_bin6/5(Mxy_In04)
  [m_xy_10] -> hist_bin6/6(Mxy_In10)
  [m_xy_23] -> hist_bin6/14(Mxy_In23)
  [m_xy_31] -> hist_bin6/17(Mxy_In31)
  [m_xy_30] -> hist_bin6/16(Mxy_In30)
  [m_xy_12] -> hist_bin6/8(Mxy_In12)
  [m_xy_32] -> hist_bin6/18(Mxy_In32)
  [m_xy_13] -> hist_bin6/9(Mxy_In13)
  [m_xy_33] -> hist_bin6/19(Mxy_In33)
  [m_xy_41] -> hist_bin6/22(Mxy_In41)
  [m_xy_01] -> hist_bin6/2(Mxy_In01)
  [m_xy_14] -> hist_bin6/10(Mxy_In14)
  [m_xy_40] -> hist_bin6/21(Mxy_In40)
  [m_xy_43] -> hist_bin6/24(Mxy_In43)
  [m_xy_20] -> hist_bin6/11(Mxy_In20)
  [m_xy_22] -> hist_bin6/13(Mxy_In22)
  [m_xy_24] -> hist_bin6/15(Mxy_In24)
  [m_xy_34] -> hist_bin6/20(Mxy_In34)
  [m_xy_03] -> hist_bin6/4(Mxy_In03)
  [m_xy_00] -> hist_bin6/1(Mxy_In00)
  [m_xy_11] -> hist_bin6/7(Mxy_In11)
  [m_xy_21] -> hist_bin6/12(Mxy_In21)
  [orien_31] -> hist_bin6/42(Orien_In31)
  [orien_34] -> hist_bin6/45(Orien_In34)
  [m_xy_42] -> hist_bin6/23(Mxy_In42)
  [orien_01] -> hist_bin6/27(Orien_In01)
  [orien_00] -> hist_bin6/26(Orien_In00)
  [orien_04] -> hist_bin6/30(Orien_In04)
  [orien_13] -> hist_bin6/34(Orien_In13)
  [orien_20] -> hist_bin6/36(Orien_In20)
  [orien_24] -> hist_bin6/40(Orien_In24)
  [orien_33] -> hist_bin6/44(Orien_In33)
  [orien_32] -> hist_bin6/43(Orien_In32)
  [orien_41] -> hist_bin6/47(Orien_In41)
  [orien_11] -> hist_bin6/32(Orien_In11)
  [orien_21] -> hist_bin6/37(Orien_In21)
  [orien_14] -> hist_bin6/35(Orien_In14)
  [orien_22] -> hist_bin6/38(Orien_In22)
  [orien_23] -> hist_bin6/39(Orien_In23)
  [orien_02] -> hist_bin6/28(Orien_In02)
  [orien_10] -> hist_bin6/31(Orien_In10)
  [orien_12] -> hist_bin6/33(Orien_In12)
  [orien_30] -> hist_bin6/41(Orien_In30)
  [m_xy_44] -> hist_bin6/25(Mxy_In44)
  [orien_03] -> hist_bin6/29(Orien_In03)
  [orien_40] -> hist_bin6/46(Orien_In40)
  [clken] -> hist_bin6/51(clken)
  hist_bin6/1(bin_out) -> [hist_bin6]
  [orien_42] -> hist_bin6/48(Orien_In42)
  [orien_44] -> hist_bin6/50(Orien_In44)
  [orien_43] -> hist_bin6/49(Orien_In43)
  Constant5/1 -> hist_bin6/52(bin_in)
  [m_xy_00] -> hist_bin5/1(Mxy_In00)
  [m_xy_04] -> hist_bin7/5(Mxy_In04)
  hist_bin7/1(bin_out) -> [hist_bin7]
  [m_xy_10] -> hist_bin7/6(Mxy_In10)
  [m_xy_13] -> hist_bin7/9(Mxy_In13)
  [m_xy_11] -> hist_bin7/7(Mxy_In11)
  [m_xy_12] -> hist_bin7/8(Mxy_In12)
  [m_xy_14] -> hist_bin7/10(Mxy_In14)
  [m_xy_22] -> hist_bin7/13(Mxy_In22)
  [m_xy_40] -> hist_bin7/21(Mxy_In40)
  [m_xy_43] -> hist_bin7/24(Mxy_In43)
  [m_xy_42] -> hist_bin7/23(Mxy_In42)
  [m_xy_44] -> hist_bin7/25(Mxy_In44)
  [m_xy_24] -> hist_bin7/15(Mxy_In24)
  [m_xy_21] -> hist_bin7/12(Mxy_In21)
  [m_xy_20] -> hist_bin7/11(Mxy_In20)
  [m_xy_23] -> hist_bin7/14(Mxy_In23)
  [m_xy_41] -> hist_bin7/22(Mxy_In41)
  [m_xy_01] -> hist_bin7/2(Mxy_In01)
  [m_xy_31] -> hist_bin7/17(Mxy_In31)
  [m_xy_30] -> hist_bin7/16(Mxy_In30)
  [m_xy_34] -> hist_bin7/20(Mxy_In34)
  [m_xy_33] -> hist_bin7/19(Mxy_In33)
  [m_xy_32] -> hist_bin7/18(Mxy_In32)
  [m_xy_03] -> hist_bin7/4(Mxy_In03)
  [m_xy_02] -> hist_bin7/3(Mxy_In02)
  [orien_10] -> hist_bin7/31(Orien_In10)
  [orien_42] -> hist_bin7/48(Orien_In42)
  [orien_01] -> hist_bin7/27(Orien_In01)
  [orien_20] -> hist_bin7/36(Orien_In20)
  [orien_31] -> hist_bin7/42(Orien_In31)
  [orien_33] -> hist_bin7/44(Orien_In33)
  [orien_21] -> hist_bin7/37(Orien_In21)
  [orien_24] -> hist_bin7/40(Orien_In24)
  [orien_03] -> hist_bin7/29(Orien_In03)
  [orien_30] -> hist_bin7/41(Orien_In30)
  [orien_12] -> hist_bin7/33(Orien_In12)
  [orien_23] -> hist_bin7/39(Orien_In23)
  [orien_32] -> hist_bin7/43(Orien_In32)
  [orien_41] -> hist_bin7/47(Orien_In41)
  [orien_43] -> hist_bin7/49(Orien_In43)
  [orien_02] -> hist_bin7/28(Orien_In02)
  [orien_00] -> hist_bin7/26(Orien_In00)
  [orien_11] -> hist_bin7/32(Orien_In11)
  [orien_34] -> hist_bin7/45(Orien_In34)
  [orien_22] -> hist_bin7/38(Orien_In22)
  [orien_04] -> hist_bin7/30(Orien_In04)
  [orien_14] -> hist_bin7/35(Orien_In14)
  [orien_44] -> hist_bin7/50(Orien_In44)
  [orien_13] -> hist_bin7/34(Orien_In13)
  [orien_40] -> hist_bin7/46(Orien_In40)
  [clken] -> hist_bin7/51(clken)
  Constant6/1 -> hist_bin7/52(bin_in)
  [m_xy_02] -> hist_bin8/3(Mxy_In02)
  [m_xy_04] -> hist_bin8/5(Mxy_In04)
  [m_xy_10] -> hist_bin8/6(Mxy_In10)
  [m_xy_23] -> hist_bin8/14(Mxy_In23)
  [m_xy_31] -> hist_bin8/17(Mxy_In31)
  [m_xy_30] -> hist_bin8/16(Mxy_In30)
  [m_xy_12] -> hist_bin8/8(Mxy_In12)
  [m_xy_32] -> hist_bin8/18(Mxy_In32)
  [m_xy_13] -> hist_bin8/9(Mxy_In13)
  [m_xy_33] -> hist_bin8/19(Mxy_In33)
  [m_xy_41] -> hist_bin8/22(Mxy_In41)
  [m_xy_01] -> hist_bin8/2(Mxy_In01)
  [m_xy_14] -> hist_bin8/10(Mxy_In14)
  [m_xy_40] -> hist_bin8/21(Mxy_In40)
  [m_xy_43] -> hist_bin8/24(Mxy_In43)
  [m_xy_20] -> hist_bin8/11(Mxy_In20)
  [m_xy_22] -> hist_bin8/13(Mxy_In22)
  [m_xy_24] -> hist_bin8/15(Mxy_In24)
  [m_xy_34] -> hist_bin8/20(Mxy_In34)
  [m_xy_03] -> hist_bin8/4(Mxy_In03)
  [m_xy_00] -> hist_bin8/1(Mxy_In00)
  [m_xy_11] -> hist_bin8/7(Mxy_In11)
  [m_xy_21] -> hist_bin8/12(Mxy_In21)
  [orien_31] -> hist_bin8/42(Orien_In31)
  [orien_34] -> hist_bin8/45(Orien_In34)
  [m_xy_42] -> hist_bin8/23(Mxy_In42)
  [orien_01] -> hist_bin8/27(Orien_In01)
  [orien_00] -> hist_bin8/26(Orien_In00)
  [orien_04] -> hist_bin8/30(Orien_In04)
  [orien_13] -> hist_bin8/34(Orien_In13)
  [orien_20] -> hist_bin8/36(Orien_In20)
  [orien_24] -> hist_bin8/40(Orien_In24)
  [orien_33] -> hist_bin8/44(Orien_In33)
  [orien_32] -> hist_bin8/43(Orien_In32)
  [orien_41] -> hist_bin8/47(Orien_In41)
  [orien_11] -> hist_bin8/32(Orien_In11)
  [orien_21] -> hist_bin8/37(Orien_In21)
  [orien_14] -> hist_bin8/35(Orien_In14)
  [orien_22] -> hist_bin8/38(Orien_In22)
  [orien_23] -> hist_bin8/39(Orien_In23)
  [orien_02] -> hist_bin8/28(Orien_In02)
  [orien_10] -> hist_bin8/31(Orien_In10)
  [orien_12] -> hist_bin8/33(Orien_In12)
  [orien_30] -> hist_bin8/41(Orien_In30)
  [m_xy_44] -> hist_bin8/25(Mxy_In44)
  [orien_03] -> hist_bin8/29(Orien_In03)
  [orien_40] -> hist_bin8/46(Orien_In40)
  [clken] -> hist_bin8/51(clken)
  hist_bin8/1(bin_out) -> [hist_bin8]
  [orien_42] -> hist_bin8/48(Orien_In42)
  [orien_44] -> hist_bin8/50(Orien_In44)
  [orien_43] -> hist_bin8/49(Orien_In43)
  Constant7/1 -> hist_bin8/52(bin_in)
  [m_xy_00] -> hist_bin7/1(Mxy_In00)
  Subsystem/1(bin1_out) -> To Workspace1/1, hist_bin1_out/1

== system test2/octave2/scale_space ==
  data_in : Inport
  valid_in : Inport  Port=2
  Gaussian_scale2 : Subsystem
  scale2 : Outport
  wires:
  data_in/1 -> [pixel_in]
  valid_in/1 -> [valid_in]
  [pixel_in] -> Gaussian_scale2/1(pixel_in)
  [valid_in] -> Gaussian_scale2/2(valid_in)
  [pixel_scale2] -> scale2/1
  Gaussian_scale2/1(pixel_out) -> [pixel_scale2]

== system test2/octave2/GradOrien/lineBuff_3x3 ==
  dataIn : Inport
  clken : Inport  Port=2
  Delay : allblocks_alteradspbuilder2/Delay  pipeline=1  pipeline_display=1  ClockPhase=1  use_ena=on  use_sclr=off  allowFloatingPointOverride=on  logOutputs=off  logFile=C:\Users\ASUS\Desktop\sift_fpga_final\Octave_2\tb_test2\test2_octave2_GradOrien_lineBuff%5F3x3_Delay.fixedpointlog  use_init=off  reset_value=1
  Delay1 : allblocks_alteradspbuilder2/Delay  pipeline=1  pipeline_display=1  ClockPhase=1  use_ena=on  use_sclr=off  allowFloatingPointOverride=on  logOutputs=off  logFile=C:\Users\ASUS\Desktop\sift_fpga_final\Octave_2\tb_test2\test2_octave2_GradOrien_lineBuff%5F3x3_Delay1.fixedpointlog  use_init=off  reset_value=1
  Delay2 : allblocks_alteradspbuilder2/Delay  pipeline=1  pipeline_display=1  ClockPhase=1  use_ena=on  use_sclr=off  allowFloatingPointOverride=on  logOutputs=off  logFile=C:\Users\ASUS\Desktop\sift_fpga_final\Octave_2\tb_test2\test2_octave2_GradOrien_lineBuff%5F3x3_Delay2.fixedpointlog  use_init=off  reset_value=1
  Delay5 : allblocks_alteradspbuilder2/Delay  pipeline=1  pipeline_display=1  ClockPhase=1  use_ena=on  use_sclr=off  allowFloatingPointOverride=on  logOutputs=off  logFile=C:\Users\ASUS\Desktop\sift_fpga_final\Octave_2\tb_test2\test2_octave2_GradOrien_lineBuff%5F3x3_Delay5.fixedpointlog  use_init=off  reset_value=1
  Delay6 : allblocks_alteradspbuilder2/Delay  pipeline=1  pipeline_display=1  ClockPhase=1  use_ena=on  use_sclr=off  allowFloatingPointOverride=on  logOutputs=off  logFile=C:\Users\ASUS\Desktop\sift_fpga_final\Octave_2\tb_test2\test2_octave2_GradOrien_lineBuff%5F3x3_Delay6.fixedpointlog  use_init=off  reset_value=1
  Delay9 : allblocks_alteradspbuilder2/Delay  pipeline=1  pipeline_display=1  ClockPhase=1  use_ena=on  use_sclr=off  allowFloatingPointOverride=on  logOutputs=off  logFile=C:\Users\ASUS\Desktop\sift_fpga_final\Octave_2\tb_test2\test2_octave2_GradOrien_lineBuff%5F3x3_Delay9.fixedpointlog  use_init=off  reset_value=1
  Memory Delay : allblocks_alteradspbuilder2/Memory Delay  BusType=Unsigned Integer  bwl=8  bwr=16  pipeline=638  pipeline_display=638  ram_type=AUTO  use_ena=on  use_sclr=off  allowFloatingPointOverride=on  logOutputs=off  logFile=C:\Users\ASUS\Desktop\sift_fpga_final\Octave_2\tb_test2\test2_octave2_GradOrien_lineBuff%5F3x3_Memory+Delay.fixedpointlog
  Memory Delay1 : allblocks_alteradspbuilder2/Memory Delay  BusType=Unsigned Fractional  bwl=8  bwr=16  pipeline=638  pipeline_display=638  ram_type=AUTO  use_ena=on  use_sclr=off  allowFloatingPointOverride=on  logOutputs=off  logFile=C:\Users\ASUS\Desktop\sift_fpga_final\Octave_2\tb_test2\test2_octave2_GradOrien_lineBuff%5F3x3_Memory+Delay1.fixedpointlog
  To Workspace : ToWorkspace  VariableName=data_in1  SaveFormat=Timeseries  SampleTime=-1
  To Workspace1 : ToWorkspace  VariableName=data_in2  SaveFormat=Timeseries  SampleTime=-1
  Out01 : Outport
  Out10 : Outport  Port=2
  Out12 : Outport  Port=3
  Out21 : Outport  Port=4
  wires:
  Delay1/1 -> [data_01], Delay2/1
  [clken] -> Memory Delay1/2
  Delay6/1 -> Memory Delay1/1, [data_12]
  Memory Delay1/1 -> Delay9/1
  [clken] -> Delay9/2
  [clken] -> Delay1/2
  [clken] -> Delay/2
  [data_in] -> To Workspace/1, Delay/1
  [clken] -> Delay2/2
  Delay2/1 -> Memory Delay/1
  clken/1 -> [clken]
  [data_21] -> Out21/1
  [data_10] -> Out10/1
  Memory Delay/1 -> [data_10], Delay5/1
  [clken] -> Memory Delay/2
  [clken] -> Delay6/2
  Delay5/1 -> Delay6/1
  [data_12] -> Out12/1
  [data_01] -> Out01/1
  [clken] -> Delay5/2
  dataIn/1 -> [data_in]
  Delay9/1 -> [data_21]
  Delay/1 -> To Workspace1/1, Delay1/1
